simulink model "Aeromobile2E"  (R2022b)
settings: Solver=VariableStepAuto  StartTime=0.0  StopTime=60  RelTol=1e-3
undefined symbols (not defined in the file or in its folder): Cc, Cis, Go
settings Model: Creator=Davide  LastModifiedBy=Davide

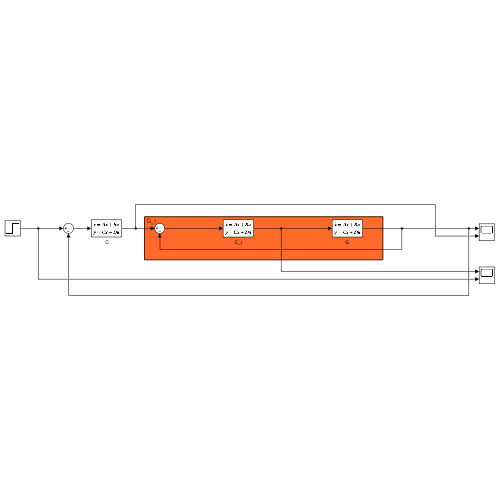
[thumbnail: Simulink's stored preview of the top-level diagram]
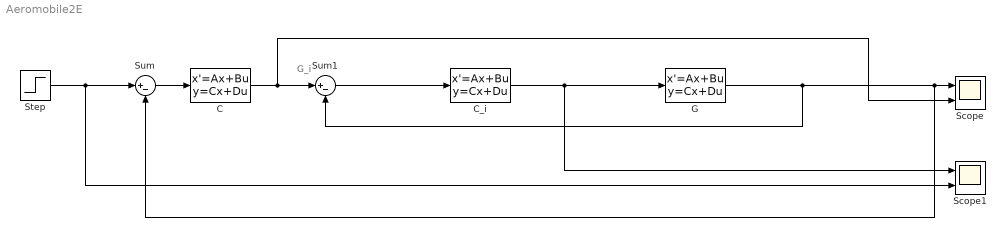
== system Aeromobile2E ==
  note: G_i
  " C" : StateSpace  A=Cc.A  B=Cc.B  C=Cc.C  D=Cc.D  InitialCondition=0
  C_i : StateSpace  A=Cis.A  B=Cis.B  C=Cis.C  D=Cis.D  InitialCondition=0
  G : StateSpace  A=Go.A  B=Go.B  C=Go.C  D=Go.D  InitialCondition=0
  Scope : Scope  NumInputPorts=2
  Scope1 : Scope  NumInputPorts=2
  Step : Step  SampleTime=0
  Sum : Sum  Inputs=|+-
  Sum1 : Sum  Inputs=|+-
  wires:
  " C"/1 -> Scope/2, Sum1/1
  G/1 -> Sum1/2, Scope/1, Sum/2
  Step/1 -> Scope1/2, Sum/1
  Sum1/1 -> C_i/1
  Sum/1 -> " C"/1
  C_i/1 -> Scope1/1, G/1
